simulink model "CryoDetHcd"  (R2016b)
settings: Solver=ode45  StartTime=0.0  StopTime=1e-3  RelTol=1e-3
PreLoadFcn:
  | setup_hcd
values from neighbouring files (symbols this model uses):
  A = sqrt(0.5*erfc(x))    [setup_hcd.m]
  Fadc = 307.2e6    (= 307200000)    [setupADCtoDACloopback.m]    (also in setupCryoFPGA_CMB.m; setup_hcd.m = 614000000)
undefined symbols (not defined in the file or in its folder): AXI4, B, C, D, etaRomData, freqRomData, freqRomData1, freqRomData2, freqRomData3, j, Lite
libraries: xbsIndex_r4 x897, CryoDetLibCMB x8, hdlsllib x8, dspsigops x2, simulink x1
(part 3 of 8)

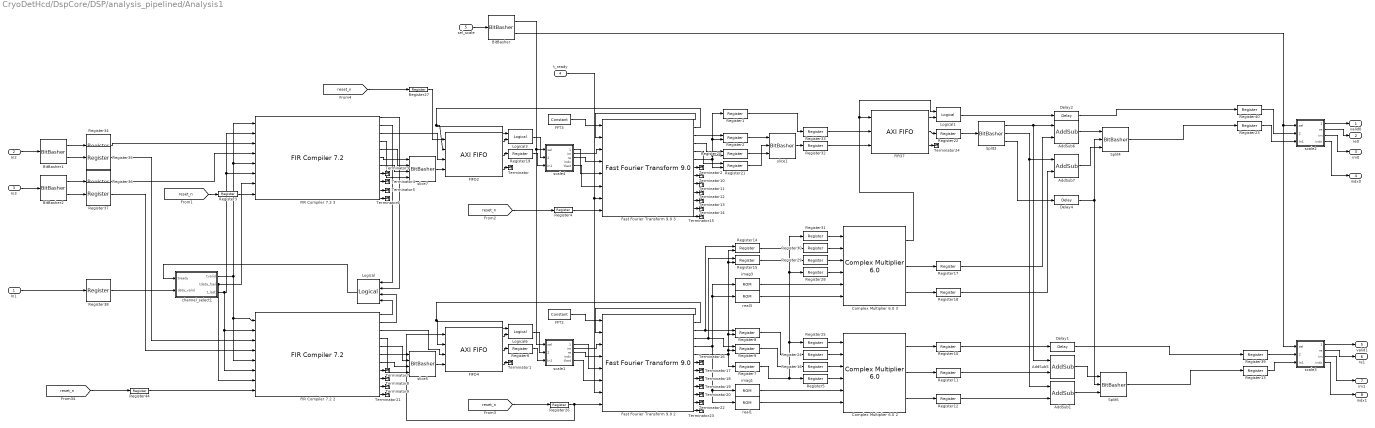
== system CryoDetHcd/DspCore/DSP/analysis_pipelined/Analysis1 ==
  In1 : Inport
  In2 : Inport  Port=2
  In3 : Inport  Port=3
  t_ready : Inport  Port=4
  sel_scale : Inport  Port=5
  AddSub{1,5..7} (4 alike) : xbsIndex_r4/AddSub  mode=Addition  use_carryin=off  use_carryout=off  en=off  latency=2  precision=Full  arith_type="Signed  (2's comp)"  n_bits=22  bin_pt=16  quantization=Truncate  overflow=Wrap  use_behavioral_HDL=on  hw_selection=Fabric  pipelined=off  dbl_ovrd=off  block_type=addsub
  BitBasher : xbsIndex_r4/BitBasher  bitexpr=|  display_expr=off  sr_1=sel0  arith_type1=Unsigned  bin_pt1=0  sr_2=sel1  arith_type2=Unsigned  bin_pt2=0  sr_3=3  arith_type3=Unsigned  bin_pt3=0  sr_4=4  arith_type4=Unsigned  bin_pt4=0  dbl_ovrd=off  block_type=bitbasher
      | sel0 = {in[0]}
      | sel1 = {in[1]}
  BitBasher1 : xbsIndex_r4/BitBasher  bitexpr=|  display_expr=off  sr_1=lo  arith_type1="Signed  (2's comp)"  bin_pt1=15  sr_2=hi  arith_type2="Signed  (2's comp)"  bin_pt2=15  sr_3=hi  arith_type3=Unsigned  bin_pt3=0  sr_4=4  arith_type4=Unsigned  bin_pt4=0  dbl_ovrd=off  block_type=bitbasher
      | lo = {in[15:0]}
      | hi = {in[31:16]}
  BitBasher2 : xbsIndex_r4/BitBasher  bitexpr=|  display_expr=off  sr_1=lo  arith_type1="Signed  (2's comp)"  bin_pt1=15  sr_2=hi  arith_type2="Signed  (2's comp)"  bin_pt2=15  sr_3=hi  arith_type3=Unsigned  bin_pt3=0  sr_4=4  arith_type4=Unsigned  bin_pt4=0  dbl_ovrd=off  block_type=bitbasher
      | lo = {in[15:0]}
      | hi = {in[31:16]}
  Complex Multiplier 6.0 2 : xbsIndex_r4/Complex Multiplier 6.0   hasatlast=off  hasatuser=off  atuserwidth=1  hasbtlast=off  hasbtuser=off  btuserwidth=1  multtype=Use_Mults  optimizegoal=Performance  flowcontrol=NonBlocking  outputwidth=24  roundmode=Truncate  hasctrltlast=off  hasctrltuser=off  ctrltuserwidth=1  outtlastbehv=Null  latencyconfig=Automatic  minimumlatency=34  aclken=off  aresetn=off  trim_axipin_name=on  simulation_type=hybrid_sim  simulation_model=sysgen:cmpy_v6_0  data_path_portlist={ 's_axis_a_tdata_real', 's_axis_a_tdata_imag', 's_axis_b_tdata_real', 's_axis_b_tdata_imag', 's_axis_ctrl_tdata_rounding_bit', 'm_axis_dout_tdata_real', 'm_axis_dout_tdata_imag' }  aportwidth=63  bportwidth=63  ip_name=Complex Multiplier  ip_version=6.0  dsptool_ready=true  ipcore_usecache=true  ipcore_useipmodelcache=true  ipcore_verbose=false  ipcore_latency_parameter='minimumlatency'  wrapper_available=true  port_translation_map={ 'aclken' => 'en', 'aresetn' => 'rst'}  block_type=cmpy_v6_0
  Complex Multiplier 6.0 3 : xbsIndex_r4/Complex Multiplier 6.0   hasatlast=off  hasatuser=off  atuserwidth=1  hasbtlast=off  hasbtuser=off  btuserwidth=1  multtype=Use_Mults  optimizegoal=Performance  flowcontrol=NonBlocking  outputwidth=24  roundmode=Truncate  hasctrltlast=off  hasctrltuser=off  ctrltuserwidth=1  outtlastbehv=Null  latencyconfig=Automatic  minimumlatency=34  aclken=off  aresetn=off  trim_axipin_name=on  simulation_type=hybrid_sim  simulation_model=sysgen:cmpy_v6_0  data_path_portlist={ 's_axis_a_tdata_real', 's_axis_a_tdata_imag', 's_axis_b_tdata_real', 's_axis_b_tdata_imag', 's_axis_ctrl_tdata_rounding_bit', 'm_axis_dout_tdata_real', 'm_axis_dout_tdata_imag' }  aportwidth=63  bportwidth=63  ip_name=Complex Multiplier  ip_version=6.0  dsptool_ready=true  ipcore_usecache=true  ipcore_useipmodelcache=true  ipcore_verbose=false  ipcore_latency_parameter='minimumlatency'  wrapper_available=true  port_translation_map={ 'aclken' => 'en', 'aresetn' => 'rst'}  block_type=cmpy_v6_0
  Delay1 : xbsIndex_r4/Delay  rst=off  infoeditControl=Selection of Reset will increase slice count due to use of real FFs and instead of SRLs  en=off  latency=2  reg_retiming=on  dbl_ovrd=off  block_type=delay
  Delay2 : xbsIndex_r4/Delay  rst=off  infoeditControl=Selection of Reset will increase slice count due to use of real FFs and instead of SRLs  en=off  latency=2  reg_retiming=on  dbl_ovrd=off  block_type=delay
  Delay4 : xbsIndex_r4/Delay  rst=off  infoeditControl=Selection of Reset will increase slice count due to use of real FFs and instead of SRLs  en=off  latency=2  reg_retiming=on  dbl_ovrd=off  block_type=delay
  FFT2 : xbsIndex_r4/Constant  const=1  gui_display_data_type=Fixed-point  arith_type=Unsigned  n_bits=1  bin_pt=0  preci_type=Single  exp_width=8  frac_width=24  explicit_period=off  period=1  equ=P=C  opselect=C  inp2=PCIN>>17  opr=+  inp1=P  carry=CIN  dbl_ovrd=off  block_type=constant
  FFT3 : xbsIndex_r4/Constant  const=1  gui_display_data_type=Fixed-point  arith_type=Unsigned  n_bits=1  bin_pt=0  preci_type=Single  exp_width=8  frac_width=24  explicit_period=off  period=1  equ=P=C  opselect=C  inp2=PCIN>>17  opr=+  inp1=P  carry=CIN  dbl_ovrd=off  block_type=constant
  FIFO2 : xbsIndex_r4/AXI FIFO  input_depth_axis=16  actual_fifo_depth_label=18  enable_tdata=on  enable_tdest=off  enable_tstrb=off  enable_tready=on  enable_tid=off  enable_tuser=off  enable_tkeep=off  enable_tlast=off  has_aresetn=on  enable_data_counts_axis=off  fifo_implementation_type_axis=Common Clock Distributed RAM  trim_axipin_name=on  programmable_full_type_axis=Full  full_threshold_assert_value_axis=0  programmable_empty_type_axis=Empty  empty_threshold_assert_value_axis=1022  underflow_flag_axi=0  underflow_sense_axi=Active High  overflow_flag_axi=0  overflow_sense_axi=Active High  block_type=axi_fifo
  FIFO4 : xbsIndex_r4/AXI FIFO  input_depth_axis=16  actual_fifo_depth_label=18  enable_tdata=on  enable_tdest=off  enable_tstrb=off  enable_tready=on  enable_tid=off  enable_tuser=off  enable_tkeep=off  enable_tlast=off  has_aresetn=on  enable_data_counts_axis=off  fifo_implementation_type_axis=Common Clock Distributed RAM  trim_axipin_name=on  programmable_full_type_axis=Full  full_threshold_assert_value_axis=0  programmable_empty_type_axis=Empty  empty_threshold_assert_value_axis=1022  underflow_flag_axi=0  underflow_sense_axi=Active High  overflow_flag_axi=0  overflow_sense_axi=Active High  block_type=axi_fifo
  FIFO7 : xbsIndex_r4/AXI FIFO  input_depth_axis=32  actual_fifo_depth_label=34  enable_tdata=on  enable_tdest=off  enable_tstrb=off  enable_tready=on  enable_tid=off  enable_tuser=off  enable_tkeep=off  enable_tlast=off  has_aresetn=off  enable_data_counts_axis=off  fifo_implementation_type_axis=Common Clock Distributed RAM  trim_axipin_name=on  programmable_full_type_axis=Full  full_threshold_assert_value_axis=0  programmable_empty_type_axis=Empty  empty_threshold_assert_value_axis=1022  underflow_flag_axi=0  underflow_sense_axi=Active High  overflow_flag_axi=0  overflow_sense_axi=Active High  block_type=axi_fifo
  FIR Compiler 7.2 2 : xbsIndex_r4/FIR Compiler 7.2   coefficientvector=analysis_coefficients2  coefficient_sets=8  coefficient_reload=off  filter_type=Single_Rate  rate_change_type=Integer  interpolation_rate=1  decimation_rate=1  zero_pack_factor=1  channel_sequence=Basic  number_channels=8  pattern_list='P4-0,P4-1,P4-2,P4-3,P4-4'  number_paths=2  ratespecification=Output_Sample_Period  sampleperiod=1.00000000  hardwareoversamplingrate=1  coefficient_sign=Signed  quantization=Quantize_Only  coefficient_width=25  bestprecision=on  coefficient_fractional_bits=28  coefficient_structure=Inferred  output_rounding_mode=Convergent_Rounding_to_Even  output_width=19  filter_architecture=Systolic_Multiply_Accumulate  optimization_goal=Area  optimization_list='None'  data_buffer_type=Automatic  coefficient_buffer_type=Automatic  input_buffer_type=Automatic  output_buffer_type=Automatic  preference_for_other_storage=Automatic  multi_column_support=Automatic  columnconfig='16'  inter_column_pipe_length=4  data_has_tlast=Vector_Framing  m_data_has_tready=off  s_data_has_fifo=off  s_data_has_tuser=Not_Required  m_data_has_tuser=Chan_ID_Field  s_config_sync_mode=On_Vector  s_config_method=By_Channel  num_reload_slots=1  has_aclken=off  has_aresetn=on  infoeditControl=ARESETn must be asserted for a minimum of 2 cycles  reset_data_vector=on  trim_axipin_name=on  simulation_type=hybrid_sim  simulation_model=sysgen:xfirv7_2_cmodel  data_path_portlist={ 's_axis_data_tdata', 'm_axis_data_tdata' }  passband_min=0.0  passband_max=0.5  stopband_min=0.5  stopband_max=1.0  filter_selection=1  gui_behaviour='Sysgen_GUI'  data_sign=Signed  data_width=16  data_fractional_bits=0  data_tuser_width=1  wrapper_available=true  ip_wrap_arbitrary_binary_point=true  ip_name=FIR Compiler  ip_version=7.2  dsptool_ready=true  ipcore_usecache=true  ipcore_useipmodelcache=true  port_translation_map={ 'aclken' => 'en', 'aresetn' => 'rst' }  run_core_at_system_period=true  ipcore_xco_need_fpga_part=true  block_type=fir_compiler_v7_2
      settings: infoedit=Maximum Possible : Maximizes oversampling rate. Abstracted input handshake (no s_data_tvalid) and automatic rate propagation.<br>Hardware Oversampling Rate : Specifies oversampling rate relative to the input sample period. Abstracted input handshake (no s_data_tvalid) and automatic rate propagation.<br>Input/Output Sample Period : Specifies absolute oversampling rate. No input handshake abstraction (exposes s_data_tvalid) and no rate propagation.
  FIR Compiler 7.2 3 : xbsIndex_r4/FIR Compiler 7.2   coefficientvector=analysis_coefficients1  coefficient_sets=8  coefficient_reload=off  filter_type=Single_Rate  rate_change_type=Integer  interpolation_rate=1  decimation_rate=1  zero_pack_factor=1  channel_sequence=Basic  number_channels=8  pattern_list='P4-0,P4-1,P4-2,P4-3,P4-4'  number_paths=2  ratespecification=Output_Sample_Period  sampleperiod=1.00000000  hardwareoversamplingrate=1  coefficient_sign=Signed  quantization=Quantize_Only  coefficient_width=25  bestprecision=on  coefficient_fractional_bits=28  coefficient_structure=Inferred  output_rounding_mode=Convergent_Rounding_to_Even  output_width=19  filter_architecture=Systolic_Multiply_Accumulate  optimization_goal=Area  optimization_list='None'  data_buffer_type=Automatic  coefficient_buffer_type=Automatic  input_buffer_type=Automatic  output_buffer_type=Automatic  preference_for_other_storage=Automatic  multi_column_support=Automatic  columnconfig='16'  inter_column_pipe_length=4  data_has_tlast=Vector_Framing  m_data_has_tready=off  s_data_has_fifo=off  s_data_has_tuser=Not_Required  m_data_has_tuser=Chan_ID_Field  s_config_sync_mode=On_Vector  s_config_method=By_Channel  num_reload_slots=1  has_aclken=off  has_aresetn=on  infoeditControl=ARESETn must be asserted for a minimum of 2 cycles  reset_data_vector=on  trim_axipin_name=on  simulation_type=hybrid_sim  simulation_model=sysgen:xfirv7_2_cmodel  data_path_portlist={ 's_axis_data_tdata', 'm_axis_data_tdata' }  passband_min=0.0  passband_max=0.5  stopband_min=0.5  stopband_max=1.0  filter_selection=1  gui_behaviour='Sysgen_GUI'  data_sign=Signed  data_width=16  data_fractional_bits=0  data_tuser_width=1  wrapper_available=true  ip_wrap_arbitrary_binary_point=true  ip_name=FIR Compiler  ip_version=7.2  dsptool_ready=true  ipcore_usecache=true  ipcore_useipmodelcache=true  port_translation_map={ 'aclken' => 'en', 'aresetn' => 'rst' }  run_core_at_system_period=true  ipcore_xco_need_fpga_part=true  block_type=fir_compiler_v7_2
      settings: infoedit=Maximum Possible : Maximizes oversampling rate. Abstracted input handshake (no s_data_tvalid) and automatic rate propagation.<br>Hardware Oversampling Rate : Specifies oversampling rate relative to the input sample period. Abstracted input handshake (no s_data_tvalid) and automatic rate propagation.<br>Input/Output Sample Period : Specifies absolute oversampling rate. No input handshake abstraction (exposes s_data_tvalid) and no rate propagation.
  Fast Fourier Transform 9.0 2 : xbsIndex_r4/Fast Fourier Transform 9.0   transform_length=8  target_clock_frequency=307  target_data_throughput=50  implementation_options=pipelined_streaming_io  run_time_configurable_transform_length=off  phase_factor_width=17  scaling_options=unscaled  rounding_modes=convergent_rounding  aclken=off  aresetn=on  output_ordering=natural_order  cyclic_prefix_insertion=off  throttle_scheme=nonrealtime  xk_index=on  ovflo=off  trim_axipin_name=on  memory_options_data=block_ram  memory_options_phase_factors=block_ram  number_of_stages_using_block_ram_for_data_and_phase_factors=0  memory_options_reorder=block_ram  memory_options_hybrid=off  complex_mult_type=use_mults_performance  butterfly_type=use_xtremedsp_slices  simulation_type=hybrid_sim  simulation_model=sysgen:xfftv9_cmodel  data_path_portlist={ 's_axis_data_tdata', 'm_axis_data_tdata', 'm_axis_status_tdata', 'event_fft_overflow' }  channels=1  input_ordering=natural_order  input_width=16  ip_name=Fast Fourier Transform  ip_version=9.0  dsptool_ready=true  ipcore_usecache=true  ipcore_useipmodelcache=true  wrapper_available=true  port_translation_map={ 'aclken' => 'en', 'aresetn' => 'rst'}  data_format=fixed_point  block_type=xfft_v9_0
  Fast Fourier Transform 9.0 3 : xbsIndex_r4/Fast Fourier Transform 9.0   transform_length=8  target_clock_frequency=307  target_data_throughput=50  implementation_options=pipelined_streaming_io  run_time_configurable_transform_length=off  phase_factor_width=17  scaling_options=unscaled  rounding_modes=convergent_rounding  aclken=off  aresetn=on  output_ordering=natural_order  cyclic_prefix_insertion=off  throttle_scheme=nonrealtime  xk_index=on  ovflo=off  trim_axipin_name=on  memory_options_data=block_ram  memory_options_phase_factors=block_ram  number_of_stages_using_block_ram_for_data_and_phase_factors=0  memory_options_reorder=block_ram  memory_options_hybrid=off  complex_mult_type=use_mults_performance  butterfly_type=use_xtremedsp_slices  simulation_type=hybrid_sim  simulation_model=sysgen:xfftv9_cmodel  data_path_portlist={ 's_axis_data_tdata', 'm_axis_data_tdata', 'm_axis_status_tdata', 'event_fft_overflow' }  channels=1  input_ordering=natural_order  input_width=16  ip_name=Fast Fourier Transform  ip_version=9.0  dsptool_ready=true  ipcore_usecache=true  ipcore_useipmodelcache=true  wrapper_available=true  port_translation_map={ 'aclken' => 'en', 'aresetn' => 'rst'}  data_format=fixed_point  block_type=xfft_v9_0
  Logical : xbsIndex_r4/Logical  logical_function=AND  inputs=4  en=off  latency=1  precision=Full  arith_type=Unsigned  n_bits=16  bin_pt=0  align_bp=on  dbl_ovrd=off  block_type=logical
  Logical1 : xbsIndex_r4/Logical  logical_function=AND  inputs=2  en=off  latency=1  precision=Full  arith_type=Unsigned  n_bits=16  bin_pt=0  align_bp=on  dbl_ovrd=off  block_type=logical
  Logical3 : xbsIndex_r4/Logical  logical_function=AND  inputs=2  en=off  latency=1  precision=Full  arith_type=Unsigned  n_bits=16  bin_pt=0  align_bp=on  dbl_ovrd=off  block_type=logical
  Logical6 : xbsIndex_r4/Logical  logical_function=AND  inputs=2  en=off  latency=1  precision=Full  arith_type=Unsigned  n_bits=16  bin_pt=0  align_bp=on  dbl_ovrd=off  block_type=logical
  Register{1,3..7,10..13,16..19,22..40,44} (34 alike) : xbsIndex_r4/Register  init=0  rst=off  en=off  dbl_ovrd=off  block_type=register
  Register{2,8..9,14..15,20..21} (7 alike) : xbsIndex_r4/Register  init=0  rst=off  en=on  dbl_ovrd=off  block_type=register
  Split3 : xbsIndex_r4/BitBasher  bitexpr=|  display_expr=off  sr_1=im  arith_type1="Signed  (2's comp)"  bin_pt1=17  sr_2=re  arith_type2="Signed  (2's comp)"  bin_pt2=17  sr_3=indx  arith_type3=Unsigned  bin_pt3=0  sr_4=4  arith_type4=Unsigned  bin_pt4=0  dbl_ovrd=off  block_type=bitbasher
      | im={in[43:22]}
      | re={in[21:0]}
      | indx = {in[46:44]}
  Split4 : xbsIndex_r4/BitBasher  bitexpr=out = {9'b0, indx, im, re}  display_expr=off  sr_1=out  arith_type1="Signed  (2's comp)"  bin_pt1=0  sr_2=im  arith_type2="Signed  (2's comp)"  bin_pt2=18  sr_3=3  arith_type3=Unsigned  bin_pt3=0  sr_4=4  arith_type4=Unsigned  bin_pt4=0  dbl_ovrd=off  block_type=bitbasher
  Split5 : xbsIndex_r4/BitBasher  bitexpr=out = {9'b0, indx, im, re}  display_expr=off  sr_1=out  arith_type1="Signed  (2's comp)"  bin_pt1=0  sr_2=im  arith_type2="Signed  (2's comp)"  bin_pt2=18  sr_3=3  arith_type3=Unsigned  bin_pt3=0  sr_4=4  arith_type4=Unsigned  bin_pt4=0  dbl_ovrd=off  block_type=bitbasher
  Terminator{,1..24} (25 alike) : Terminator
  channel_select1 : Subsystem
  imag1 : xbsIndex_r4/ROM  depth=8  initVector=imag(exp(-j*2*pi*(8:15)/16))  distributed_mem=Block RAM  rst=off  init_reg=0  en=off  latency=2  gui_display_data_type=Fixed-point  arith_type="Signed  (2's comp)"  n_bits=18  bin_pt=16  preci_type=Single  exp_width=8  frac_width=24  optimize=Area  use_rpm=on  dbl_ovrd=off  block_type=sprom
  imag3 : xbsIndex_r4/ROM  depth=8  initVector=imag(exp(-j*2*pi*(0:7)/16))  distributed_mem=Block RAM  rst=off  init_reg=0  en=off  latency=2  gui_display_data_type=Fixed-point  arith_type="Signed  (2's comp)"  n_bits=18  bin_pt=16  preci_type=Single  exp_width=8  frac_width=24  optimize=Area  use_rpm=on  dbl_ovrd=off  block_type=sprom
  real1 : xbsIndex_r4/ROM  depth=8  initVector=real(exp(-j*2*pi*(8:15)/16))  distributed_mem=Block RAM  rst=off  init_reg=0  en=off  latency=2  gui_display_data_type=Fixed-point  arith_type="Signed  (2's comp)"  n_bits=18  bin_pt=16  preci_type=Single  exp_width=8  frac_width=24  optimize=Area  use_rpm=on  dbl_ovrd=off  block_type=sprom
  real3 : xbsIndex_r4/ROM  depth=8  initVector=real(exp(-j*2*pi*(0:7)/16))  distributed_mem=Block RAM  rst=off  init_reg=0  en=off  latency=2  gui_display_data_type=Fixed-point  arith_type="Signed  (2's comp)"  n_bits=18  bin_pt=16  preci_type=Single  exp_width=8  frac_width=24  optimize=Area  use_rpm=on  dbl_ovrd=off  block_type=sprom
  scale1 : Subsystem
  scale2 : Subsystem
  scale3 : Subsystem
  scale4 : Subsystem
  slice1 : xbsIndex_r4/BitBasher  bitexpr="out ={17'b0,  indx, im, re }"  display_expr=off  sr_1=out  arith_type1=Unsigned  bin_pt1=0  sr_2=2  arith_type2="Signed  (2's comp)"  bin_pt2=16  sr_3=3  arith_type3=Unsigned  bin_pt3=0  sr_4=4  arith_type4=Unsigned  bin_pt4=0  dbl_ovrd=off  block_type=bitbasher
  slice5 : xbsIndex_r4/BitBasher  bitexpr=out ={19'b0, tlast, indx, im[20:0], re[20:0] }  display_expr=off  sr_1=out  arith_type1=Unsigned  bin_pt1=0  sr_2=2  arith_type2="Signed  (2's comp)"  bin_pt2=16  sr_3=3  arith_type3=Unsigned  bin_pt3=0  sr_4=4  arith_type4=Unsigned  bin_pt4=0  dbl_ovrd=off  block_type=bitbasher
  slice7 : xbsIndex_r4/BitBasher  bitexpr=out ={19'b0, tlast, indx, im[20:0], re[20:0] }  display_expr=off  sr_1=out  arith_type1=Unsigned  bin_pt1=0  sr_2=2  arith_type2="Signed  (2's comp)"  bin_pt2=16  sr_3=3  arith_type3=Unsigned  bin_pt3=0  sr_4=4  arith_type4=Unsigned  bin_pt4=0  dbl_ovrd=off  block_type=bitbasher
  valid0 : Outport
  re0 : Outport  Port=2
  im0 : Outport  Port=3
  indx0 : Outport  Port=4
  valid1 : Outport  Port=5
  re1 : Outport  Port=6
  im1 : Outport  Port=7
  indx1 : Outport  Port=8
  wires:
  t_ready/1 -> Fast Fourier Transform 9.0 3/7, Fast Fourier Transform 9.0 2/7
  Delay1/1 -> Register39/1
  FIR Compiler 7.2 2/3 -> FIFO4/3
  slice5/1 -> FIFO4/4
  Register27/1 -> FIFO2/1
  [reset_n] -> Register27/1
  FIR Compiler 7.2 3/3 -> FIFO2/3
  slice7/1 -> FIFO2/4
  Register26/1 -> Fast Fourier Transform 9.0 2/8, FIFO4/1
  Register4/1 -> Fast Fourier Transform 9.0 3/8
  Register3/1 -> FIR Compiler 7.2 3/8
  Register44/1 -> FIR Compiler 7.2 2/8
  [reset_n] -> Register26/1
  [reset_n] -> Register4/1
  [reset_n] -> Register3/1
  [reset_n] -> Register44/1
  BitBasher/1 -> scale4/1(sel), scale1/1(sel)
  sel_scale/1 -> BitBasher/1
  scale3/4(indx) -> indx1/1
  scale3/3(im) -> im1/1
  scale3/2(re) -> re1/1
  scale3/1(valid_o) -> valid1/1
  Register13/1 -> scale3/3(In1)
  Register39/1 -> scale3/2(valid_i)
  scale2/1(valid_o) -> valid0/1
  Register23/1 -> scale2/3(In1)
  scale2/3(im) -> im0/1
  BitBasher/2 -> scale3/1(sel), scale2/1(sel)
  scale1/3(re) -> Fast Fourier Transform 9.0 2/4
  scale1/2(im) -> Fast Fourier Transform 9.0 2/3
  scale1/1(valid_o) -> Fast Fourier Transform 9.0 2/5
  scale1/5(tlast) -> Fast Fourier Transform 9.0 2/6
  Logical3/1 -> scale4/2(valid_i)
  scale4/1(valid_o) -> Fast Fourier Transform 9.0 3/5
  scale4/2(im) -> Fast Fourier Transform 9.0 3/3
  scale4/3(re) -> Fast Fourier Transform 9.0 3/4
  BitBasher2/2 -> Register37/1
  BitBasher2/1 -> Register36/1
  BitBasher1/2 -> Register35/1
  BitBasher1/1 -> Register34/1
  Register38/1 -> channel_select1/2(data_valid)
  Register37/1 -> FIR Compiler 7.2 2/4
  Register36/1 -> FIR Compiler 7.2 3/4
  Register35/1 -> FIR Compiler 7.2 2/3
  Register34/1 -> FIR Compiler 7.2 3/3
  In2/1 -> BitBasher1/1
  Register31/1 -> Complex Multiplier 6.0 3/1
  Register30/1 -> Complex Multiplier 6.0 3/2
  Register29/1 -> Complex Multiplier 6.0 3/3
  Register28/1 -> Complex Multiplier 6.0 3/4
  imag3/1 -> Complex Multiplier 6.0 3/5
  real3/1 -> Complex Multiplier 6.0 3/6
  Register25/1 -> Complex Multiplier 6.0 2/1
  Register24/1 -> Complex Multiplier 6.0 2/2
  Register16/1 -> Complex Multiplier 6.0 2/3
  Register5/1 -> Complex Multiplier 6.0 2/4
  imag1/1 -> Complex Multiplier 6.0 2/5
  real1/1 -> Complex Multiplier 6.0 2/6
  FIR Compiler 7.2 2/6 -> slice5/1
  Fast Fourier Transform 9.0 2/5 -> imag3/1, real3/1, imag1/1, real1/1
  FIFO2/1 -> Logical3/2
  FIFO7/3 -> Terminator24/1
  Fast Fourier Transform 9.0 2/13 -> Terminator23/1
  Fast Fourier Transform 9.0 2/12 -> Terminator22/1
  Fast Fourier Transform 9.0 2/11 -> Terminator20/1
  Fast Fourier Transform 9.0 2/10 -> Terminator19/1
  Fast Fourier Transform 9.0 2/9 -> Terminator18/1
  Fast Fourier Transform 9.0 2/8 -> Terminator17/1
  Fast Fourier Transform 9.0 2/7 -> Terminator16/1
  Fast Fourier Transform 9.0 3/13 -> Terminator15/1
  Fast Fourier Transform 9.0 3/12 -> Terminator14/1
  Fast Fourier Transform 9.0 3/11 -> Terminator13/1
  Fast Fourier Transform 9.0 3/10 -> Terminator12/1
  Fast Fourier Transform 9.0 3/9 -> Terminator11/1
  Fast Fourier Transform 9.0 3/8 -> Terminator10/1
  Fast Fourier Transform 9.0 3/7 -> Terminator2/1
  FIFO4/3 -> Terminator1/1
  FIFO2/3 -> Terminator/1
  Split3/3 -> Delay4/1
  Split4/1 -> Register23/1
  scale2/4(indx) -> indx0/1
  scale2/2(re) -> re0/1
  Register40/1 -> scale2/2(valid_i)
  Delay2/1 -> Register40/1
  AddSub7/1 -> Split4/3
  AddSub6/1 -> Split4/1
  Delay4/1 -> Split4/2, Split5/2
  Logical1/1 -> Delay2/1
  Register18/1 -> AddSub7/2
  Register17/1 -> AddSub6/2
  Split3/2 -> AddSub7/1, AddSub1/1
  Split3/1 -> AddSub6/1, AddSub5/1
  Register22/1 -> Split3/1
  FIFO7/1 -> Logical1/2
  FIFO7/2 -> Register22/1
  slice1/1 -> Register32/1
  Register1/1 -> Register33/1
  Register20/1 -> slice1/3
  Register21/1 -> slice1/2
  Register2/1 -> slice1/1
  Fast Fourier Transform 9.0 3/5 -> Register21/1
  Fast Fourier Transform 9.0 3/6 -> Register21/2, Register20/2, Register2/2, Register1/1
  Fast Fourier Transform 9.0 3/4 -> Register20/1
  Fast Fourier Transform 9.0 3/3 -> Register2/1
  channel_select1/3(t_last) -> FIR Compiler 7.2 2/2, FIR Compiler 7.2 2/6, FIR Compiler 7.2 3/6, FIR Compiler 7.2 3/2
  scale4/5(tlast) -> Fast Fourier Transform 9.0 3/6
  Fast Fourier Transform 9.0 3/1 -> Fast Fourier Transform 9.0 3/2
  FFT3/1 -> Fast Fourier Transform 9.0 3/1
  Register19/1 -> scale4/3(In1)
  FIFO2/2 -> Register19/1
  Fast Fourier Transform 9.0 3/2 -> Logical3/1, FIFO2/2
  FIR Compiler 7.2 2/11 -> Terminator21/1
  FIR Compiler 7.2 2/10 -> Terminator9/1
  FIR Compiler 7.2 2/9 -> Terminator8/1
  FIR Compiler 7.2 2/8 -> Terminator7/1
  FIR Compiler 7.2 3/11 -> Terminator6/1
  FIR Compiler 7.2 3/10 -> Terminator5/1
  FIR Compiler 7.2 3/9 -> Terminator4/1
  FIR Compiler 7.2 3/8 -> Terminator3/1
  FIR Compiler 7.2 3/4 -> slice7/4
  FIR Compiler 7.2 3/5 -> slice7/2
  FIR Compiler 7.2 3/7 -> slice7/3
  FIR Compiler 7.2 3/6 -> slice7/1
  FIR Compiler 7.2 3/2 -> Logical/1
  FIR Compiler 7.2 3/1 -> Logical/2
  FIR Compiler 7.2 2/2 -> Logical/3
  FIR Compiler 7.2 2/1 -> Logical/4
  Complex Multiplier 6.0 3/3 -> Register18/1
  Complex Multiplier 6.0 3/2 -> Register17/1
  Complex Multiplier 6.0 3/1 -> FIFO7/1, Logical1/1
  Register14/1 -> Register30/1
  Register15/1 -> Register29/1
  Split5/1 -> Register13/1
  AddSub1/1 -> Split5/3
  AddSub5/1 -> Split5/1
  Register10/1 -> Delay1/1
  Register11/1 -> AddSub5/2
  Register12/1 -> AddSub1/2
  Complex Multiplier 6.0 2/1 -> Register10/1
  Complex Multiplier 6.0 2/2 -> Register11/1
  Complex Multiplier 6.0 2/3 -> Register12/1
  Register7/1 -> Register5/1, Register25/1, Register31/1, Register28/1
  Register8/1 -> Register24/1
  Register9/1 -> Register16/1
  Fast Fourier Transform 9.0 2/6 -> Register7/1, Register9/2, Register15/2, Register14/2, Register8/2
  Fast Fourier Transform 9.0 2/4 -> Register9/1, Register15/1
  Fast Fourier Transform 9.0 2/3 -> Register8/1, Register14/1
  Fast Fourier Transform 9.0 2/1 -> Fast Fourier Transform 9.0 2/2
  FFT2/1 -> Fast Fourier Transform 9.0 2/1
  FIR Compiler 7.2 2/4 -> slice5/4
  Logical6/1 -> scale1/2(valid_i)
  Register6/1 -> scale1/3(In1)
  FIFO4/2 -> Register6/1
  Fast Fourier Transform 9.0 2/2 -> Logical6/1, FIFO4/2
  FIFO4/1 -> Logical6/2
  FIR Compiler 7.2 2/5 -> slice5/2
  FIR Compiler 7.2 2/7 -> slice5/3
  Logical/1 -> channel_select1/1(tready)
  In1/1 -> Register38/1
  In3/1 -> BitBasher2/1
  channel_select1/1(tvalid) -> FIR Compiler 7.2 2/1, FIR Compiler 7.2 2/5, FIR Compiler 7.2 3/1, FIR Compiler 7.2 3/5
  channel_select1/2(tdata_fsel) -> FIR Compiler 7.2 3/7, FIR Compiler 7.2 2/7
  Register32/1 -> FIFO7/3
  Register33/1 -> FIFO7/2

== system CryoDetHcd/DspCore/DSP/analysis_pipelined/Enabled Subsystem ==
  In1 : Inport
  Enable : EnablePort
  Buffer : Buffer  N=8  TreatMby1Signals=One channel  OutputFrames=off
  Out1 : Outport
  wires:
  In1/1 -> Buffer/1
  Buffer/1 -> Out1/1

== system CryoDetHcd/DspCore/DSP/analysis_pipelined/Pre-Analysis0 ==
  valid : Inport
  im : Inport  Port=2
  re : Inport  Port=3
  Delay : xbsIndex_r4/Delay  rst=off  infoeditControl=Selection of Reset will increase slice count due to use of real FFs and instead of SRLs  en=off  latency=8  reg_retiming=on  dbl_ovrd=off  block_type=delay
  Delay1 : xbsIndex_r4/Delay  rst=off  infoeditControl=Selection of Reset will increase slice count due to use of real FFs and instead of SRLs  en=off  latency=8  reg_retiming=on  dbl_ovrd=off  block_type=delay
  Delay2 : xbsIndex_r4/Delay  rst=off  infoeditControl=Selection of Reset will increase slice count due to use of real FFs and instead of SRLs  en=off  latency=8  reg_retiming=on  dbl_ovrd=off  block_type=delay
  valid0 : Outport
  im0 : Outport  Port=2
  reo : Outport  Port=3
  wires:
  Delay2/1 -> reo/1
  Delay1/1 -> im0/1
  Delay/1 -> valid0/1
  re/1 -> Delay2/1
  im/1 -> Delay1/1
  valid/1 -> Delay/1

== system CryoDetHcd/DspCore/DSP/analysis_pipelined/Pre-Analysis1 ==
  valid : Inport
  im : Inport  Port=2
  re : Inport  Port=3
  BitBasher1 : xbsIndex_r4/BitBasher  bitexpr=|  display_expr=off  sr_1=lo  arith_type1="Signed  (2's comp)"  bin_pt1=15  sr_2=hi  arith_type2="Signed  (2's comp)"  bin_pt2=15  sr_3=hi  arith_type3=Unsigned  bin_pt3=0  sr_4=4  arith_type4=Unsigned  bin_pt4=0  dbl_ovrd=off  block_type=bitbasher
      | lo = {in[15:0]}
      | hi = {in[31:16]}
  BitBasher2 : xbsIndex_r4/BitBasher  bitexpr=out = {hi, lo}  display_expr=off  sr_1=out  arith_type1=Unsigned  bin_pt1=0  sr_2=hi  arith_type2="Signed  (2's comp)"  bin_pt2=15  sr_3=hi  arith_type3=Unsigned  bin_pt3=0  sr_4=4  arith_type4=Unsigned  bin_pt4=0  dbl_ovrd=off  block_type=bitbasher
  BitBasher3 : xbsIndex_r4/BitBasher  bitexpr=out = {hi, lo}  display_expr=off  sr_1=out  arith_type1=Unsigned  bin_pt1=0  sr_2=hi  arith_type2="Signed  (2's comp)"  bin_pt2=15  sr_3=hi  arith_type3=Unsigned  bin_pt3=0  sr_4=4  arith_type4=Unsigned  bin_pt4=0  dbl_ovrd=off  block_type=bitbasher
  BitBasher4 : xbsIndex_r4/BitBasher  bitexpr=|  display_expr=off  sr_1=lo  arith_type1="Signed  (2's comp)"  bin_pt1=15  sr_2=hi  arith_type2="Signed  (2's comp)"  bin_pt2=15  sr_3=hi  arith_type3=Unsigned  bin_pt3=0  sr_4=4  arith_type4=Unsigned  bin_pt4=0  dbl_ovrd=off  block_type=bitbasher
      | lo = {in[15:0]}
      | hi = {in[31:16]}
  "Complex Multiplier 6.0 " : xbsIndex_r4/Complex Multiplier 6.0   hasatlast=off  hasatuser=off  atuserwidth=1  hasbtlast=off  hasbtuser=off  btuserwidth=1  multtype=Use_Mults  optimizegoal=Resources  flowcontrol=NonBlocking  outputwidth=19  roundmode=Truncate  hasctrltlast=off  hasctrltuser=off  ctrltuserwidth=1  outtlastbehv=Null  latencyconfig=Automatic  minimumlatency=37  aclken=off  aresetn=off  trim_axipin_name=on  simulation_type=hybrid_sim  simulation_model=sysgen:cmpy_v6_0  data_path_portlist={ 's_axis_a_tdata_real', 's_axis_a_tdata_imag', 's_axis_b_tdata_real', 's_axis_b_tdata_imag', 's_axis_ctrl_tdata_rounding_bit', 'm_axis_dout_tdata_real', 'm_axis_dout_tdata_imag' }  aportwidth=63  bportwidth=63  ip_name=Complex Multiplier  ip_version=6.0  dsptool_ready=true  ipcore_usecache=true  ipcore_useipmodelcache=true  ipcore_verbose=false  ipcore_latency_parameter='minimumlatency'  wrapper_available=true  port_translation_map={ 'aclken' => 'en', 'aresetn' => 'rst'}  block_type=cmpy_v6_0
  Complex Multiplier 6.0 1 : xbsIndex_r4/Complex Multiplier 6.0   hasatlast=off  hasatuser=off  atuserwidth=1  hasbtlast=off  hasbtuser=off  btuserwidth=1  multtype=Use_Mults  optimizegoal=Resources  flowcontrol=NonBlocking  outputwidth=19  roundmode=Truncate  hasctrltlast=off  hasctrltuser=off  ctrltuserwidth=1  outtlastbehv=Null  latencyconfig=Automatic  minimumlatency=37  aclken=off  aresetn=off  trim_axipin_name=on  simulation_type=hybrid_sim  simulation_model=sysgen:cmpy_v6_0  data_path_portlist={ 's_axis_a_tdata_real', 's_axis_a_tdata_imag', 's_axis_b_tdata_real', 's_axis_b_tdata_imag', 's_axis_ctrl_tdata_rounding_bit', 'm_axis_dout_tdata_real', 'm_axis_dout_tdata_imag' }  aportwidth=63  bportwidth=63  ip_name=Complex Multiplier  ip_version=6.0  dsptool_ready=true  ipcore_usecache=true  ipcore_useipmodelcache=true  ipcore_verbose=false  ipcore_latency_parameter='minimumlatency'  wrapper_available=true  port_translation_map={ 'aclken' => 'en', 'aresetn' => 'rst'}  block_type=cmpy_v6_0
  Convert{,1..3} (4 alike) : xbsIndex_r4/Convert  gui_display_data_type=Fixed-point  arith_type="Signed  (2's comp)"  n_bits=16  bin_pt=15  float_type=Single  exp_bits=8  fraction_bits=24  quantization=Truncate  overflow=Flag as error  en=off  latency=0  pipeline=off  dbl_ovrd=off  block_type=convert
  Counter : xbsIndex_r4/Counter  cnt_type=Free Running  cnt_to=Inf  operation=Up  start_count=0  cnt_by_val=1  arith_type=Unsigned  n_bits=4  bin_pt=0  load_pin=off  rst=on  en=on  explicit_period=on  period=2/Fadc  use_behavioral_HDL=off  implementation=Fabric  dbl_ovrd=off  block_type=counter
  Register{,1..9,44} (11 alike) : xbsIndex_r4/Register  init=0  rst=off  en=off  dbl_ovrd=off  block_type=register
  imag1 : xbsIndex_r4/ROM  depth=16  initVector=imag(exp(-j*2*pi*(1:2:31)/32))  distributed_mem=Block RAM  rst=off  init_reg=0  en=off  latency=2  gui_display_data_type=Fixed-point  arith_type="Signed  (2's comp)"  n_bits=18  bin_pt=16  preci_type=Single  exp_width=8  frac_width=24  optimize=Area  use_rpm=on  dbl_ovrd=off  block_type=sprom
  imag2 : xbsIndex_r4/ROM  depth=16  initVector=imag(exp(-j*2*pi*(0:2:31)/32))  distributed_mem=Block RAM  rst=off  init_reg=0  en=off  latency=2  gui_display_data_type=Fixed-point  arith_type="Signed  (2's comp)"  n_bits=18  bin_pt=16  preci_type=Single  exp_width=8  frac_width=24  optimize=Area  use_rpm=on  dbl_ovrd=off  block_type=sprom
  real1 : xbsIndex_r4/ROM  depth=16  initVector=real(exp(-j*2*pi*(1:2:31)/32))  distributed_mem=Block RAM  rst=off  init_reg=0  en=off  latency=2  gui_display_data_type=Fixed-point  arith_type="Signed  (2's comp)"  n_bits=18  bin_pt=16  preci_type=Single  exp_width=8  frac_width=24  optimize=Area  use_rpm=on  dbl_ovrd=off  block_type=sprom
  real2 : xbsIndex_r4/ROM  depth=16  initVector=real(exp(-j*2*pi*(0:2:31)/32))  distributed_mem=Block RAM  rst=off  init_reg=0  en=off  latency=2  gui_display_data_type=Fixed-point  arith_type="Signed  (2's comp)"  n_bits=18  bin_pt=16  preci_type=Single  exp_width=8  frac_width=24  optimize=Area  use_rpm=on  dbl_ovrd=off  block_type=sprom
  valid0 : Outport
  im0 : Outport  Port=2
  reo : Outport  Port=3
  wires:
  real1/1 -> Complex Multiplier 6.0 1/6
  imag1/1 -> Complex Multiplier 6.0 1/5
  Register7/1 -> Complex Multiplier 6.0 1/3
  Register6/1 -> Complex Multiplier 6.0 1/2
  real2/1 -> "Complex Multiplier 6.0 "/6
  imag2/1 -> "Complex Multiplier 6.0 "/5
  Register3/1 -> "Complex Multiplier 6.0 "/3
  Register2/1 -> "Complex Multiplier 6.0 "/2
  Register1/1 -> "Complex Multiplier 6.0 "/1, Complex Multiplier 6.0 1/4, Complex Multiplier 6.0 1/1, "Complex Multiplier 6.0 "/4
  BitBasher4/1 -> Register5/1
  Convert1/1 -> BitBasher2/2
  "Complex Multiplier 6.0 "/1 -> valid0/1
  Register/1 -> Register1/1
  Convert3/1 -> BitBasher3/2
  Convert2/1 -> BitBasher3/1
  Convert/1 -> BitBasher2/1
  valid/1 -> Counter/2, Register/1
  BitBasher3/1 -> reo/1
  BitBasher2/1 -> im0/1
  Counter/1 -> real1/1, imag1/1, real2/1, imag2/1
  BitBasher4/2 -> Register9/1
  BitBasher1/2 -> Register8/1
  BitBasher1/1 -> Register4/1
  re/1 -> BitBasher4/1
  im/1 -> BitBasher1/1
  Register4/1 -> Register2/1
  Register5/1 -> Register3/1
  Register8/1 -> Register6/1
  Register9/1 -> Register7/1
  Complex Multiplier 6.0 1/2 -> Convert/1
  "Complex Multiplier 6.0 "/2 -> Convert1/1
  Complex Multiplier 6.0 1/3 -> Convert2/1
  "Complex Multiplier 6.0 "/3 -> Convert3/1
  [reset] -> Register44/1
  Register44/1 -> Counter/1

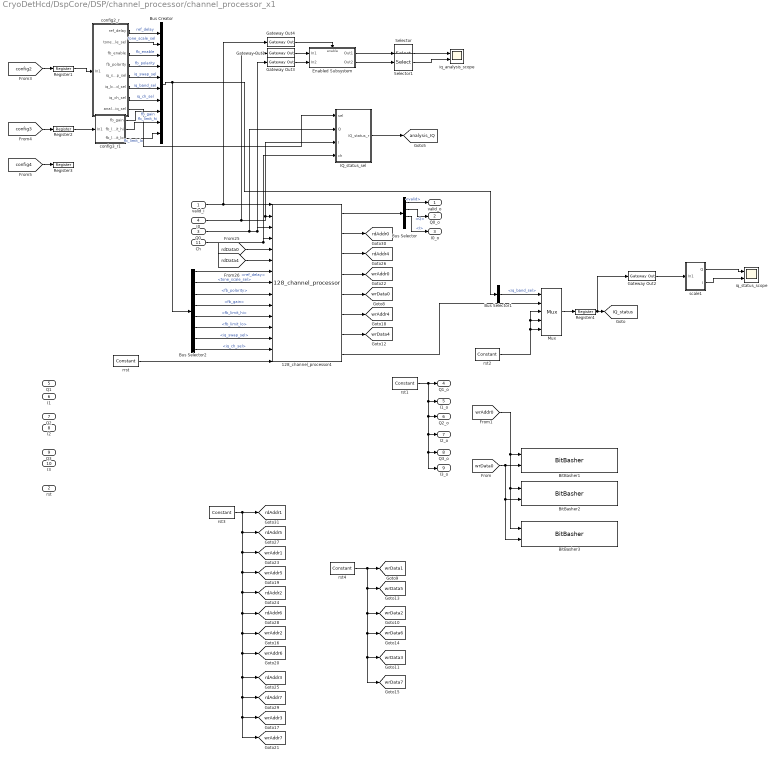
== system CryoDetHcd/DspCore/DSP/channel_processor/channel_processor_x1 ==
  valid_i : Inport
  rst : Inport  Port=2
  Q0 : Inport  Port=3
  I0 : Inport  Port=4
  Q1 : Inport  Port=5
  I1 : Inport  Port=6
  Q2 : Inport  Port=7
  I2 : Inport  Port=8
  Q3 : Inport  Port=9
  I3 : Inport  Port=10
  Ch : Inport  Port=11
  128_channel_processor4 : CryoDetLibCMB/128_channel_processor
  BitBasher1 : xbsIndex_r4/BitBasher  bitexpr=out = {2'b01, ch, freq[23:1]}  display_expr=on  sr_1=out  arith_type1=Unsigned  bin_pt1=0  sr_2=2  arith_type2=Unsigned  bin_pt2=0  sr_3=3  arith_type3=Unsigned  bin_pt3=0  sr_4=4  arith_type4=Unsigned  bin_pt4=0  dbl_ovrd=off  block_type=bitbasher
  BitBasher2 : xbsIndex_r4/BitBasher  bitexpr=out = {2'b10, ch, freq[23:1]}  display_expr=on  sr_1=out  arith_type1=Unsigned  bin_pt1=0  sr_2=2  arith_type2=Unsigned  bin_pt2=0  sr_3=3  arith_type3=Unsigned  bin_pt3=0  sr_4=4  arith_type4=Unsigned  bin_pt4=0  dbl_ovrd=off  block_type=bitbasher
  BitBasher3 : xbsIndex_r4/BitBasher  bitexpr=out = {2'b11, ch, freq[23:1]}  display_expr=on  sr_1=out  arith_type1=Unsigned  bin_pt1=0  sr_2=2  arith_type2=Unsigned  bin_pt2=0  sr_3=3  arith_type3=Unsigned  bin_pt3=0  sr_4=4  arith_type4=Unsigned  bin_pt4=0  dbl_ovrd=off  block_type=bitbasher
  Bus Creator : BusCreator  Inputs=10
  Bus Selector : BusSelector  OutputSignals=valid,Q,I,ch
  Bus Selector1 : BusSelector  OutputSignals=iq_band_sel
  Bus Selector2 : BusSelector  OutputSignals=ref_delay,tone_scale_sel,fb_polarity,fb_gain,fb_limit_hi,fb_limit_lo,iq_swap_sel,iq_ch_sel
  Enabled Subsystem : Subsystem  TreatAsAtomicUnit=on
  Gateway Out{1..4} (4 alike) : xbsIndex_r4/Gateway Out  inherit_from_input=on  hdl_port=off  rows=1  columns=1  UseAsDAC=off  DACChannel='1'  interface=None  automatic_assignment=on  address_offset=hex2dec('00')  intf_name=''  intf_description=''  timing_constraint=None  locs_specified=off  LOCs={}  io_standard={}  block_type=gatewayout
  IQ_status_sel : Subsystem
  Mux : xbsIndex_r4/Mux  inputs=4  en=off  latency=1  precision=Full  arith_type=Unsigned  n_bits=16  bin_pt=14  quantization=Truncate  overflow=Wrap  dbl_ovrd=off  block_type=mux
  Register{1..4} (4 alike) : xbsIndex_r4/Register  init=0  rst=off  en=off  dbl_ovrd=off  block_type=register
  Selector : Selector  InputPortWidth=8  IndexOptions=Index vector (dialog)  Indices=[1]  OutputSizes=1
  Selector1 : Selector  InputPortWidth=8  IndexOptions=Index vector (dialog)  Indices=[1]  OutputSizes=1
  config2_r : Subsystem  AncestorBlock=CryoDetLibCMB/config2_r
  config3_r1 : Subsystem  AncestorBlock=CryoDetLibCMB/config3_r
  iq_analysis_scope : Scope  NumInputPorts=2
  iq_status_scope : Scope  NumInputPorts=2
  rrst : xbsIndex_r4/Constant  const=0  gui_display_data_type=Fixed-point  arith_type=Unsigned  n_bits=1  bin_pt=0  preci_type=Single  exp_width=8  frac_width=24  explicit_period=on  period=2/Fadc  equ=P=C  opselect=C  inp2=PCIN>>17  opr=+  inp1=P  carry=CIN  dbl_ovrd=off  block_type=constant
  rst1 : xbsIndex_r4/Constant  const=0  gui_display_data_type=Fixed-point  arith_type=Signed (2's comp)  n_bits=16  bin_pt=15  preci_type=Single  exp_width=8  frac_width=24  explicit_period=on  period=2/Fadc  equ=P=C  opselect=C  inp2=PCIN>>17  opr=+  inp1=P  carry=CIN  dbl_ovrd=off  block_type=constant
  rst2 : xbsIndex_r4/Constant  const=0  gui_display_data_type=Fixed-point  arith_type=Unsigned  n_bits=32  bin_pt=0  preci_type=Single  exp_width=8  frac_width=24  explicit_period=on  period=2/Fadc  equ=P=C  opselect=C  inp2=PCIN>>17  opr=+  inp1=P  carry=CIN  dbl_ovrd=off  block_type=constant
  rst3 : xbsIndex_r4/Constant  const=0  gui_display_data_type=Fixed-point  arith_type=Unsigned  n_bits=7  bin_pt=0  preci_type=Single  exp_width=8  frac_width=24  explicit_period=on  period=2/Fadc  equ=P=C  opselect=C  inp2=PCIN>>17  opr=+  inp1=P  carry=CIN  dbl_ovrd=off  block_type=constant
  rst4 : xbsIndex_r4/Constant  const=0  gui_display_data_type=Fixed-point  arith_type=Unsigned  n_bits=32  bin_pt=0  preci_type=Single  exp_width=8  frac_width=24  explicit_period=on  period=2/Fadc  equ=P=C  opselect=C  inp2=PCIN>>17  opr=+  inp1=P  carry=CIN  dbl_ovrd=off  block_type=constant
  scale1 : Subsystem
  valid_o : Outport
  Q0_o : Outport  Port=2
  I0_o : Outport  Port=3
  Q1_o : Outport  Port=4
  I1_o : Outport  Port=5
  Q2_o : Outport  Port=6
  I2_o : Outport  Port=7
  Q3_o : Outport  Port=8
  I3_o : Outport  Port=9
  tag scope: IQ_status=global, analysis_IQ=global, rdAddr0=global, rdAddr1=global, rdAddr2=global, rdAddr3=global, rdAddr4=global, rdAddr5=global, rdAddr6=global, rdAddr7=global, wrAddr0=global, wrAddr1=global, wrAddr2=global, wrAddr3=global, wrAddr4=global, wrAddr5=global, wrAddr6=global, wrAddr7=global, wrData0=global, wrData1=global, wrData2=global, wrData3=global, wrData4=global, wrData5=global, wrData6=global, wrData7=global
  wires:
  128_channel_processor4/3 -> [rdAddr4]
  128_channel_processor4/2 -> [rdAddr0]
  128_channel_processor4/6 -> [wrAddr4]
  128_channel_processor4/4 -> [wrAddr0]
  128_channel_processor4/5 -> [wrData0]
  128_channel_processor4/7 -> [wrData4]
  [rdData0] -> 128_channel_processor4/5
  [rdData4] -> 128_channel_processor4/6
  Ch/1 -> IQ_status_sel/4(ch), 128_channel_processor4/4
  I0/1 -> Gateway Out1/1, IQ_status_sel/3(I), 128_channel_processor4/2
  Q0/1 -> IQ_status_sel/2(Q), Gateway Out3/1, 128_channel_processor4/3
  valid_i/1 -> 128_channel_processor4/1, Gateway Out4/1
  128_channel_processor4/1 -> Bus Selector/1
  Bus Selector/2 -> Q0_o/1  "<Q>"
  Bus Selector/3 -> I0_o/1  "<I>"
  [config2] -> Register1/1
  [config3] -> Register2/1
  [config4] -> Register3/1
  Register2/1 -> config3_r1/1(In1)
  Bus Selector/1 -> valid_o/1  "<valid>"
  Register1/1 -> config2_r/1(In1)
  Mux/1 -> Register4/1
  Register4/1 -> Gateway Out2/1, [IQ_status]
  128_channel_processor4/8 -> Mux/2
  rst1/1 -> I1_o/1, Q2_o/1, I2_o/1, I3_o/1, Q3_o/1, Q1_o/1
  rst2/1 -> Mux/4, Mux/3, Mux/5
  rst4/1 -> [wrData5], [wrData2], [wrData6], [wrData3], [wrData7], [wrData1]
  rst3/1 -> [rdAddr5], [wrAddr1], [wrAddr5], [rdAddr2], [rdAddr6], [wrAddr2], [wrAddr6], [rdAddr3], [rdAddr7], [wrAddr3], [wrAddr7], [rdAddr1]
  config2_r/5(iq_swap_sel) -> Bus Creator/5  "iq_swap_sel"
  config2_r/7(iq_ch_sel) -> Bus Creator/7  "iq_ch_sel"
  config2_r/6(iq_band_sel) -> Bus Creator/6  "iq_band_sel"
  config2_r/1(ref_delay) -> Bus Creator/1  "ref_delay"
  config2_r/2(tone_scale_sel) -> Bus Creator/2  "tone_scale_sel"
  config2_r/3(fb_enable) -> Bus Creator/3  "fb_enable"
  config2_r/4(fb_polarity) -> Bus Creator/4  "fb_polarity"
  Bus Creator/1 -> Bus Selector2/1, Bus Selector1/1
  Bus Selector1/1 -> Mux/1  "<iq_band_sel>"
  [wrAddr0] -> BitBasher1/1, BitBasher3/1, BitBasher2/1
  [wrData0] -> BitBasher1/2, BitBasher3/2, BitBasher2/2
  Gateway Out2/1 -> scale1/1(In1)
  scale1/1(Q) -> iq_status_scope/1
  scale1/2(I) -> iq_status_scope/2
  Enabled Subsystem/2(Out2) -> Selector1/1
  Enabled Subsystem/1(Out1) -> Selector/1
  Selector1/1 -> iq_analysis_scope/2
  Selector/1 -> iq_analysis_scope/1
  Gateway Out1/1 -> Enabled Subsystem/1(In1)
  Gateway Out3/1 -> Enabled Subsystem/2(In2)
  Gateway Out4/1 -> Enabled Subsystem/Enable
  config2_r/8(analysis_iq_sel) -> IQ_status_sel/1(sel)
  IQ_status_sel/1(IQ_status_r) -> [analysis_IQ]
  config3_r1/3(fb_limit_lo) -> Bus Creator/10  "fb_limit_lo"
  config3_r1/2(fb_limit_hi) -> Bus Creator/9  "fb_limit_hi"
  config3_r1/1(fb_gain) -> Bus Creator/8  "fb_gain"
  Bus Selector2/4 -> 128_channel_processor4/10  "<fb_gain>"
  Bus Selector2/5 -> 128_channel_processor4/11  "<fb_limit_hi>"
  Bus Selector2/3 -> 128_channel_processor4/9  "<fb_polarity>"
  Bus Selector2/6 -> 128_channel_processor4/12  "<fb_limit_lo>"
  Bus Selector2/2 -> 128_channel_processor4/8  "<tone_scale_sel>"
  Bus Selector2/1 -> 128_channel_processor4/7  "<ref_delay>"
  Bus Selector2/7 -> 128_channel_processor4/13  "<iq_swap_sel>"
  Bus Selector2/8 -> 128_channel_processor4/14  "<iq_ch_sel>"
  rrst/1 -> 128_channel_processor4/15
